simulink model "reverb"  (R2016a)
settings: Solver=VariableStepAuto  StartTime=0.0  StopTime=10.0  RelTol=1e-3
libraries: dspsrcs4 x1
settings Model: Creator=joa-m  LastModifiedBy=joa-m

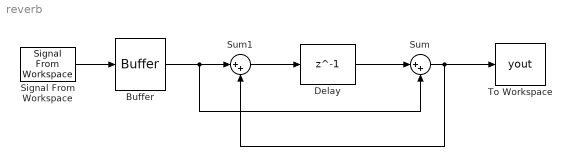
== system reverb ==
  Buffer : Buffer  N=1  TreatMby1Signals=One channel  OutputFrames=off
  Delay : Delay  DelayLength=1  InputProcessing=Columns as channels (frame based)
  Signal From Workspace : dspsrcs4/Signal From Workspace  X=[1,2,0,3]  Ts=1  nsamps=1  OutputAfterFinalValue=Setting to zero  ignoreOrWarnInputAndFrameLengths=off  OutputFrames=off
  Sum : Sum  Inputs=|++
  Sum1 : Sum  Inputs=|++
  To Workspace : ToWorkspace  VariableName=yout  SampleTime=-1
      settings: Save2DSignal=2-D array (concatenate along first dimension)
  wires:
  Delay/1 -> Sum/1
  Sum/1 -> To Workspace/1, Sum1/2
  Sum1/1 -> Delay/1
  Buffer/1 -> Sum/2, Sum1/1
  Signal From Workspace/1 -> Buffer/1
